simulink model "servoModel"  (R2023b)
settings: Solver=FixedStepAuto  StartTime=0.0  StopTime=50  FixedStep=1e-4  RelTol=1e-3
values from neighbouring files (symbols this model uses):
  k = (1/2) * sqrt((Ps - Pr + PL_at_x0)/(Ps - Pr - PL_at_x0)) - 1    [myCode.m]    (also in servoData_Final.mat = 1.82709080211)
  K = (sqrt(2) * Q_max) / (sqrt(DeltaP_FlowGain) * I_max)    [myCode.m]    (also in servoData_Final.mat = 3.34485685962e-06)
  m3Ps2lpm = 1/ lpm2m3Ps    (= 60000)    [myCode.m]    (also in servoData_Final.mat)
  Pa2Bar = 1/1e5    (= 1e-05)    [myCode.m]    (also in servoData_Final.mat)
  Ps = 2980 * psi2Pa    (= 20546376.7242)    [myCode.m]    (also in servoData_Final.mat)
  x0 = Qs_at_x0 / (sqrt(2)*K*sqrt(Ps - Pr))    [myCode.m]    (also in servoData_Final.mat = 0.000534280669171)
undefined symbols (not defined in the file or in its folder): AEFF, B_E, L_STROKE, V01, V02
libraries: simulink x1
settings Model: Creator=snr  LastModifiedBy=snr

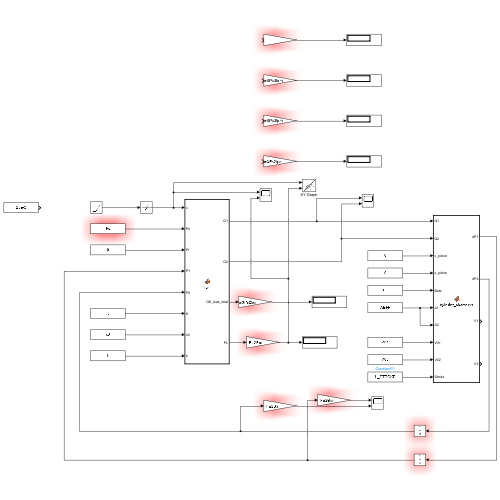
[thumbnail: Simulink's stored preview of the top-level diagram]
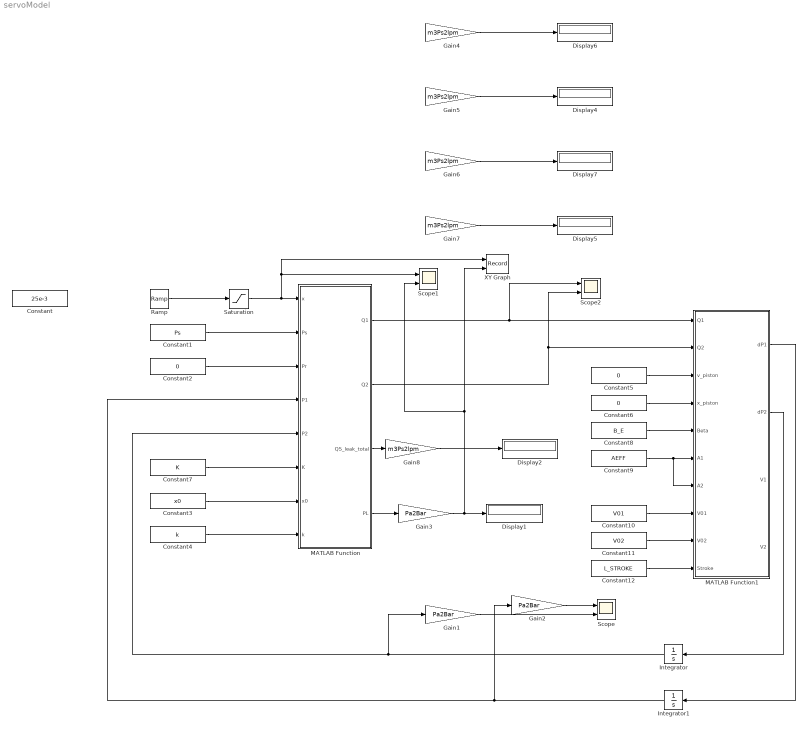
== system servoModel ==
  Constant : Constant  Value=25e-3
  Constant1 : Constant  Value=Ps
  Constant10 : Constant  Value=V01
  Constant11 : Constant  Value=V02
  Constant12 : Constant  Value=L_STROKE
  Constant2 : Constant  Value=0
  Constant3 : Constant  Value=x0
  Constant4 : Constant  Value=k
  Constant5 : Constant  Value=0
  Constant6 : Constant  Value=0
  Constant7 : Constant  Value=K
  Constant8 : Constant  Value=B_E
  Constant9 : Constant  Value=AEFF
  Display{1..2,4..7} (6 alike) : Display
  Gain1 : Gain  Gain=Pa2Bar
  Gain2 : Gain  Gain=Pa2Bar
  Gain3 : Gain  Gain=Pa2Bar
  Gain{4..8} (5 alike) : Gain  Gain=m3Ps2lpm
  Integrator : Integrator  InitialCondition=Ps/2
  Integrator1 : Integrator  InitialCondition=Ps/2
  MATLAB Function : MATLAB Function  TreatAsAtomicUnit=on
  MATLAB Function1 : MATLAB Function  TreatAsAtomicUnit=on
  Ramp : simulink/Sources/Ramp  slope=0.001  start=0  InitialOutput=-25e-3
  Saturation : Saturate  UpperLimit=25e-3  LowerLimit=-25e-3
  Scope : Scope  NumInputPorts=2
  Scope1 : Scope  NumInputPorts=2
  Scope2 : Scope  NumInputPorts=2
  XY Graph : Record  FileSettingsInternal="{\"entries\":[{\"content\":{\"excelSettings\":{\"content\":{},\"type\":\"Streamout.ExcelSettings\"}},\"type\":\"Streamout.FileSettingStorage\",\"uuid\":\"\"}],\"packageUris\":[\"http:\\/\\/schema.mathworks.com\\/mf0\\/streamout_blocks\\/R2020a\"],\"version\":\"1.0\"}"  Layout=[1 1]  SignalsInternal="{\"entries\":[{\"content\":{\"signals\":[{\"content\":{\"blockPath\":[],\"dimensions\":[1],\"domain\":\"\",\"lineColor\":\"#a2142f\",\"plots\":[1],\"port\":1,\"signalID\":24854,\"signalName\":\"Saturation\"},\"type\":\"RecordBlkView.Signal\",\"uuid\":\"\"},{\"content\":{\"blockPath\":[],\"dimensions\":[1],\"domain\":\"\",\"lineColor\":\"#139fff\",\"plots\":[1],\"port\":2,\"signalID\":24857,\"signalName\":\"Gain3\"},\"type\":\"RecordBlkView.Signal\",\"uuid\":\"\"}]},\"type\":\"RecordBlkView.InputSignals\",\"uuid\":\"\"}],\"packageUris\":[\"http:\\/\\/schema.mathworks.com\\/mf0\\/streamout_blocks\\/R2020a\"],\"version\":\"1.0\"}"  VisualizationBindings="{\"xyplotplugin\":{\"info\":[{\"series\":[{\"bindingParametersList\":[{\"parameter\":\"X-Axis\",\"signalID\":24854,\"signalName\":\"Saturation\"},{\"parameter\":\"Y-Axis\",\"signalID\":24857,\"signalName\":\"Gain3\"}],\"seriesID\":22055}],\"subplotID\":1}]}}"  CompatibilityTag=XY
  wires:
  Constant1/1 -> MATLAB Function/2(Ps)
  Constant7/1 -> MATLAB Function/6(K)
  Constant4/1 -> MATLAB Function/8(k)
  Constant3/1 -> MATLAB Function/7(x0)
  Constant2/1 -> MATLAB Function/3(Pr)
  Gain4/1 -> Display6/1
  Gain5/1 -> Display4/1
  Gain6/1 -> Display7/1
  Gain7/1 -> Display5/1
  MATLAB Function/1(Q1) -> Scope2/1, MATLAB Function1/1(Q1)
  MATLAB Function/2(Q2) -> Scope2/2, MATLAB Function1/2(Q2)
  Constant5/1 -> MATLAB Function1/3(v_piston)
  Constant8/1 -> MATLAB Function1/5(Beta)
  Constant9/1 -> MATLAB Function1/7(A2), MATLAB Function1/6(A1)
  Constant10/1 -> MATLAB Function1/8(V01)
  Constant11/1 -> MATLAB Function1/9(V02)
  Constant12/1 -> MATLAB Function1/10(Stroke)
  MATLAB Function1/2(dP2) -> Integrator/1
  MATLAB Function1/1(dP1) -> Integrator1/1
  Integrator/1 -> Gain1/1, MATLAB Function/5(P2)
  Gain1/1 -> Scope/2
  Gain2/1 -> Scope/1
  Integrator1/1 -> Gain2/1, MATLAB Function/4(P1)
  MATLAB Function/4(PL) -> Gain3/1
  Gain3/1 -> Scope1/2, XY Graph/2, Display1/1
  Ramp/1 -> Saturation/1
  Constant6/1 -> MATLAB Function1/4(x_piston)
  Saturation/1 -> XY Graph/1, Scope1/1, MATLAB Function/1(x)
  MATLAB Function/3(QS_leak_total) -> Gain8/1
  Gain8/1 -> Display2/1

== matlab function servoModel/MATLAB Function1 ==
  data: dP1 output; dP2 output; Q1 input; V1 output; Q2 input; v_piston input; x_piston input; Beta input; A1 input; A2 input; V01 input; V2 output; V02 input; Stroke input
function [dP1, dP2, V1, V2] = cylinder_chambers(Q1, Q2, v_piston, x_piston, Beta, A1, A2, V01, V02, Stroke)
    % GİRİŞLER:
    % Q1, Q2    : Valften gelen debiler (m^3/s) [Valve bloğunun çıkışı]
    % v_piston  : Piston hızı (m/s) [Mekanik sistemden gelecek]
    % x_piston  : Piston konumu (m) [Mekanik sistemden gelecek]
    % Beta      : Bulk Modulus (Pa) [Örn: 1.4e9]
    % A1, A2    : Piston alanları (m^2)
    % V01, V02  : Boru ve ölü hacimler (m^3)
    % Stroke    : Silindir strok boyu (m)

    % 1. ANLIK HACİMLERİN HESAPLANMASI
    % Piston ileri gittikçe (x artarsa), V1 artar, V2 azalır.
    % Güvenlik: Hacim asla 0 veya negatif olmamalı (bölme hatası olmasın diye min sınır)
    
    V1_calc = V01 + A1 * x_piston;
    V2_calc = V02 + A2 *(Stroke - x_piston);
    
    V1 = max(V1_calc, 1e-5); % Çok küçük bir minimum hacim limiti
    V2 = max(V2_calc, 1e-5);

    % 2. BASINÇ TÜREVLERİNİN HESAPLANMASI (dP/dt)
    
    % Odacık 1 (Arka Taraf):
    % Hacim genişliyor (- A1*v), İçeri Q1 giriyor.
    dP1 = (Beta / V1) * (Q1 - (A1 * v_piston));
    
    % Odacık 2 (Ön/Rod Tarafı):
    % Hacim daralıyor (+ A2*v), İçeri Q2 giriyor (veya çıkıyor).
    % Not: Piston ileri giderken (v>0) V2 küçülür, bu basıncı artırıcı etkidir.
    dP2 = (Beta / V2) * (Q2 + (A2 * v_piston));
    
end

== matlab function servoModel/MATLAB Function ==
  data: Q1 output; Q2 output; x input; QS_leak_total output; Ps input; Pr input; P1 input; P2 input; K input; x0 input; k input; PL output
function [Q1, Q2, QS_leak_total, PL] = fcn(x, Ps, Pr, P1, P2, K, x0, k)
    % Not: Girişlerden Q_tare parametresini kaldırdık.
    % Onun yerine içeride sabit K_tare tanımladık.
    
    % --- SABİT DEĞERLER ---
    % 0.64 lpm @ 3000 psi referansına göre hesaplanan katsayı:
    K_tare = 2.345e-9; 

    % --- GÜVENLİK ---
    % Basınç farklarının negatif olmamasını garanti edelim (sqrt hatası için)
    dPs1 = max(0, Ps - P1);
    dP1r = max(0, P1 - Pr);
    dPs2 = max(0, Ps - P2);
    dP2r = max(0, P2 - Pr);
    dPsr = max(0, Ps - Pr); % Pilot/Tare hattı için

    % --- ANA AKIŞ VE SPOOL SIZINTISI (MAKALE MODELİ) ---
    if x >= 0
        % P_S -> P_1 (Supply'dan 1'e akış)
        Q1_S = K * sqrt(dPs1) * (x0 + x); 
        % P_1 -> P_R (Sızıntı)
        Q1_R = K * sqrt(dP1r) * (x0^2 / (x0 + k*x)); 

        % P_S -> P_2 (Sızıntı)
        Q2_S = K * sqrt(dPs2) * (x0^2 / (x0 + k*x)); 
        % P_2 -> P_R (2'den Return'e akış)
        Q2_R = K * sqrt(dP2r) * (x0 + x); 
    else
        % x < 0 durumu
		
        Q1_S = K * sqrt(dPs1) * (x0^2 / (x0 - k*x)); % (Sızıntı)
        Q1_R = K * sqrt(dP1r) * (x0 - x);  %(1'den Return'e akış)
		
        Q2_S = K * sqrt(dPs2) * (x0 - x); %(Supply'dan 2'ye akış)
        Q2_R = K * sqrt(dP2r) * (x0^2 / (x0 - k*x)); % (Sızıntı)
    end

    % --- ÇIKIŞLAR ---
    % Portlardaki Net Akışlar
    Q1 = Q1_S - Q1_R;
    Q2 = Q2_S - Q2_R;
    
    % Yük Basıncı
    PL = P1 - P2;

    % --- TOPLAM BESLEME AKIŞI (SIZINTI HESABI) ---
    % 1. Spool üzerindeki aktif sızıntı/akış
    QS_spool = Q1_S + Q2_S; 
    
    % 2. Dinamik "Sabit" Sızıntı (Tare Leakage)
    % Basınca bağımlı hale getirildi:
    Q_tare_dynamic = K_tare * sqrt(dPsr);
    
    % Toplam
    QS_leak_total = QS_spool + Q_tare_dynamic;
end
